simulink model "cart_pend"  (R2019a)
settings: Solver=FixedStepAuto  StartTime=0.0  StopTime=30  FixedStep=0.001  RelTol=1e-3
values from neighbouring files (symbols this model uses):
  h = animatedline(road_x, road_y,'Color',[0.4660, 0.6740, 0.1880],'LineWidth',3)    [animation.m]    (also in prepare_sim.m = params.h)
  r = 10    [prepare_sim.m]
  theta0 = 0.1    [prepare_sim.m]
  thetadot0 = 0    [prepare_sim.m]
  x0 = 0    [prepare_sim.m]
  xdot0 = 0    [prepare_sim.m]
undefined symbols (not defined in the file or in its folder): params, xf
settings Model: Creator=Piku  LastModifiedBy=Piku

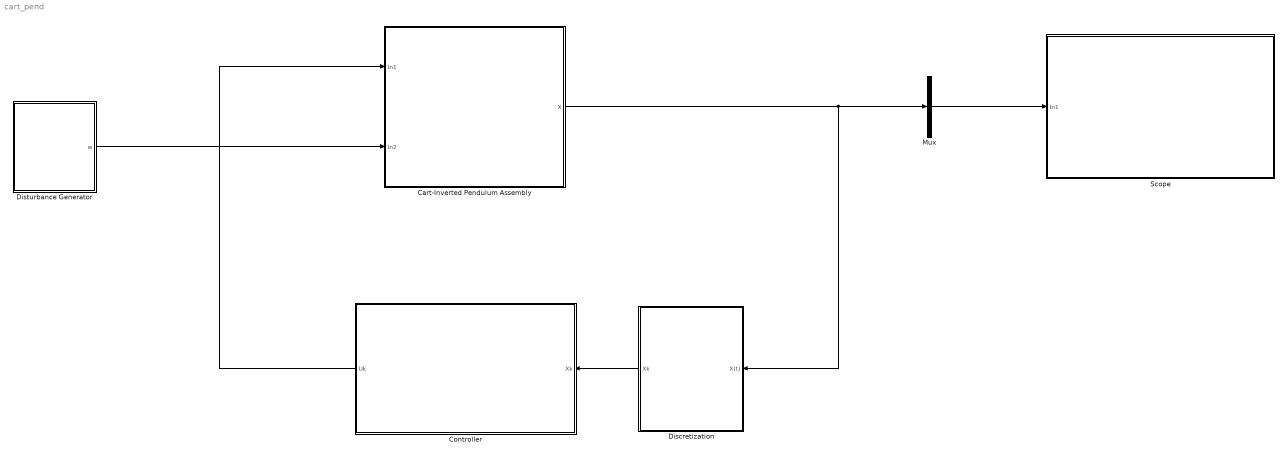
== system cart_pend ==
  Cart-Inverted Pendulum Assembly : Subsystem
      mask Display: image('cart_pendulum.png');
  Controller : Subsystem
  Discretization : Subsystem
  Disturbance Generator : Subsystem
  Mux : Mux  Inputs=1
  Scope : Subsystem
  wires:
  Cart-Inverted Pendulum Assembly/1("X ") -> Mux/1, Discretization/1(X(t))
  Controller/1(Uk) -> Cart-Inverted Pendulum Assembly/1(In1)
  Discretization/1(Xk) -> Controller/1(" Xk")
  Disturbance Generator/1(w) -> Cart-Inverted Pendulum Assembly/2(In2)
  Mux/1 -> Scope/1(In1)

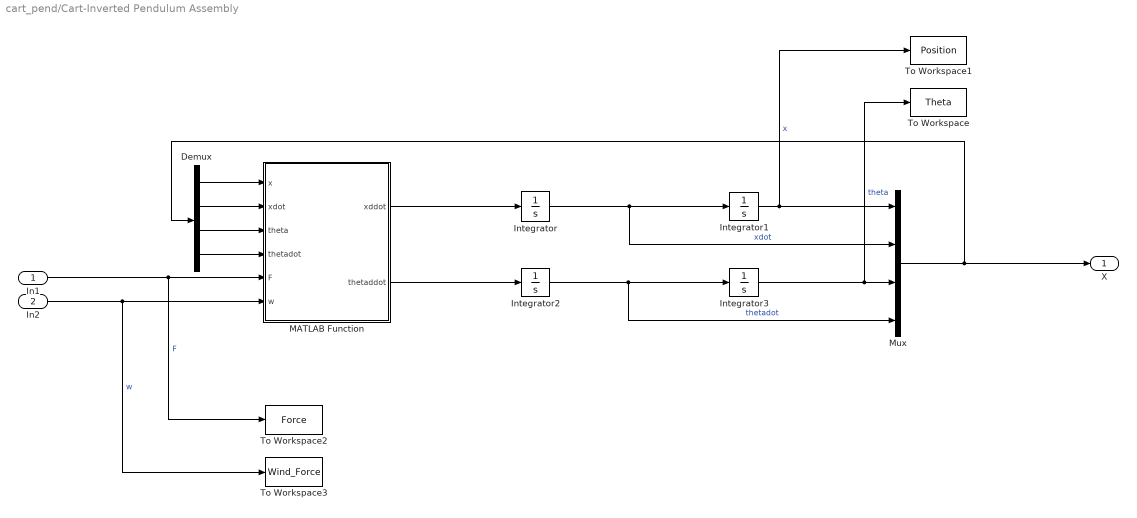
== system cart_pend/Cart-Inverted Pendulum Assembly ==
  In1 : Inport
  In2 : Inport  Port=2  PortDimensions=1
  Demux : Demux
  Integrator : Integrator  InitialCondition=xdot0  LimitOutput=on  UpperSaturationLimit=1e6  LowerSaturationLimit=-1e6
  Integrator1 : Integrator  InitialCondition=x0  UpperSaturationLimit=xf  LowerSaturationLimit=-x0
  Integrator2 : Integrator  InitialCondition=thetadot0  LimitOutput=on  UpperSaturationLimit=1e6  LowerSaturationLimit=-1e6
  Integrator3 : Integrator  InitialCondition=theta0  LimitOutput=on  UpperSaturationLimit=pi  LowerSaturationLimit=-pi
  MATLAB Function : MATLAB Function  TreatAsAtomicUnit=on
  Mux : Mux
  To Workspace : ToWorkspace  VariableName=Theta  SaveFormat=Timeseries  SampleTime=h
  To Workspace1 : ToWorkspace  VariableName=Position  SaveFormat=Timeseries  SampleTime=h
  To Workspace2 : ToWorkspace  VariableName=Force  SaveFormat=Timeseries  SampleTime=h
  To Workspace3 : ToWorkspace  VariableName=Wind_Force  SaveFormat=Timeseries  SampleTime=h
  "X " : Outport  PortDimensions=4
  wires:
  Integrator2/1 -> Integrator3/1, Mux/4  "thetadot"
  In1/1 -> To Workspace2/1, MATLAB Function/5(F)  "F"
  Integrator3/1 -> To Workspace/1, Mux/3  "theta"
  Integrator/1 -> Mux/2, Integrator1/1  "xdot"
  Integrator1/1 -> To Workspace1/1, Mux/1  "x"
  Mux/1 -> Demux/1, "X "/1
  MATLAB Function/1(xddot) -> Integrator/1
  MATLAB Function/2(thetaddot) -> Integrator2/1
  Demux/1 -> MATLAB Function/1(x)
  Demux/2 -> MATLAB Function/2(xdot)
  Demux/3 -> MATLAB Function/3(theta)
  Demux/4 -> MATLAB Function/4(thetadot)
  In2/1 -> To Workspace3/1, MATLAB Function/6(w)  "w"

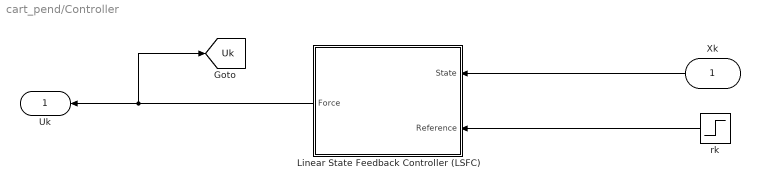
== system cart_pend/Controller ==
  " Xk" : Inport  PortDimensions=4  SampleTime=h
  Linear State Feedback Controller (LSFC) : Subsystem
  rk : Step  Time=0  Before=x0  After=r  SampleTime=h
  Uk : Outport  SampleTime=h
  tag scope: Uk=global
  wires:
  rk/1 -> Linear State Feedback Controller (LSFC)/2(Reference)
  " Xk"/1 -> Linear State Feedback Controller (LSFC)/1(State)
  Linear State Feedback Controller (LSFC)/1(Force) -> [Uk], Uk/1

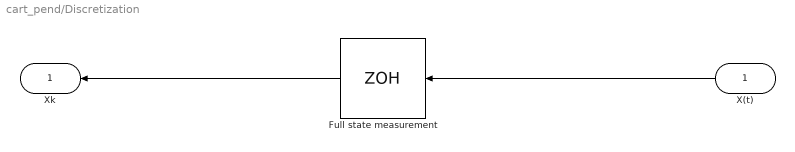
== system cart_pend/Discretization ==
  X(t) : Inport
  Full state measurement : ZeroOrderHold  SampleTime=h
  Xk : Outport  SampleTime=h
  wires:
  X(t)/1 -> Full state measurement/1
  Full state measurement/1 -> Xk/1

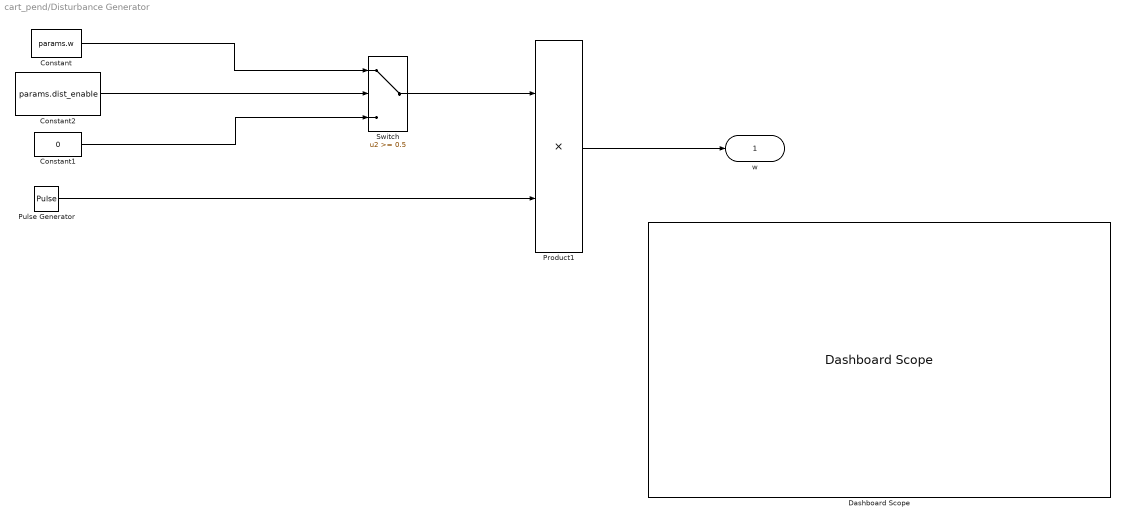
== system cart_pend/Disturbance Generator ==
  Constant : Constant  Value=params.w
  Constant1 : Constant  Value=0
  Constant2 : Constant  Value=params.dist_enable
  Dashboard Scope : DashboardScope  Ymin=0  Ymax=0.02
  Product1 : Product
  Pulse Generator : DiscretePulseGenerator  PulseType=Time based  Period=35  PulseWidth=75  PhaseDelay=15
  Switch : Switch  Threshold=0.5
  w : Outport
  wires:
  Constant2/1 -> Switch/2
  Constant1/1 -> Switch/3
  Constant/1 -> Switch/1
  Switch/1 -> Product1/1
  Product1/1 -> w/1
  Pulse Generator/1 -> Product1/2

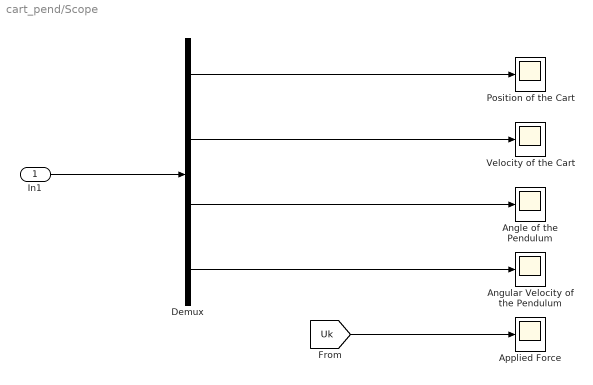
== system cart_pend/Scope ==
  In1 : Inport
  Angle of the Pendulum : Scope
  Angular Velocity of the Pendulum : Scope
  Applied Force : Scope
  Demux : Demux
  Position of the Cart : Scope
  Velocity of the Cart : Scope
  wires:
  In1/1 -> Demux/1
  Demux/1 -> Position of the Cart/1
  Demux/2 -> Velocity of the Cart/1
  Demux/3 -> Angle of the Pendulum/1
  Demux/4 -> Angular Velocity of the Pendulum/1
  [Uk] -> Applied Force/1

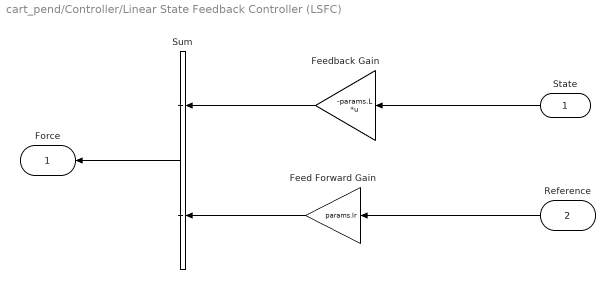
== system cart_pend/Controller/Linear State Feedback Controller (LSFC) ==
  State : Inport  PortDimensions=4  SampleTime=h
  Reference : Inport  Port=2  PortDimensions=1  SampleTime=h
  Feed Forward Gain : Gain  Gain=params.lr
  Feedback Gain : Gain  Gain=-params.L  Multiplication=Matrix(K*u) (u vector)
  Sum : Sum
  Force : Outport  SampleTime=h
  wires:
  Feed Forward Gain/1 -> Sum/2
  State/1 -> Feedback Gain/1
  Reference/1 -> Feed Forward Gain/1
  Sum/1 -> Force/1
  Feedback Gain/1 -> Sum/1

== matlab function cart_pend/Cart-Inverted Pendulum Assembly/MATLAB Function ==
  data: x input; xddot output; xdot input; theta input; thetadot input; F input; thetaddot output; w input
function [xddot, thetaddot] = fcn(x, xdot, theta, thetadot, F, w)

M   = 0.5;          % Mass of the cart      
m   = 0.2;          % Mass of the inverted pendulum
bc  = 0.1;          % coefficient of friction for cart
l   = 0.3;          % length to the pendulum center of mass
I   = 0.006;        % moment of inertia of the pendulum
bp  = 0.012;        % coefficient of friction for pendulum
g   = 9.8;          % acceleration due to gravity

% Dynamics of the pendulum
ap0 = (I + m*l^2);
ap1 = -(m^2*l^2)/(M+m);
bp0 = (m*l)/(M+m);
bp1 = 0.5*(m^2*l^2)/(M+m);
bp2 = (m*l*bc)/(M+m);
bp3 = bp;
bp4 = -m*g*l; 
bp5 = -l;
thetaddot = (1/(ap0 + ap1*cos(theta)^2))* ( bp0*cos(theta)*(F - w) ...
             - bp1*thetadot^2*sin(2*theta) - bp2*cos(theta)*xdot ...
             - bp3*thetadot - bp4*sin(theta) - bp5*cos(theta)*w );

% Dynamics of the cart
ac0 = M + m;
ac1 = - m^2*l^2/(I + m*l^2);
bc0 = 1;
bc1 = m*l;
bc2 = bc;
bc3 = (bp*m*l)/(I + m*l^2);
bc4 = -0.5*(m^2*l^2*g)/(I + m*l^2);
bc5 = -(m*l^2)/(I + m*l^2);
xddot = (1/(ac0 + ac1*cos(theta)^2))* (bc0*(F - w)...
             - bc1*thetadot^2*sin(theta) - bc2*xdot ...
             - bc3*thetadot*cos(theta) - bc4*sin(2*theta) ...
             - bc5*w*cos(theta)^2 );
end
